simulink model "reactorBlock_Simulink_Simscape_Full_Controller"  (R2023a)
settings: Solver=ode15s  StartTime=0.0  StopTime=300  FixedStep=0.1  RelTol=1e-3
libraries: nesl_utility x30, fl_lib x28, slpidlib x4, simulink x4, RankineCycle_lib x3
(part 2 of 2)

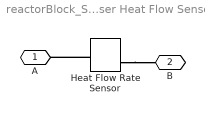
== system reactorBlock_Simulink_Simscape_Full_Controller/Condenser Heat Flow Sensor ==
  Heat Flow Rate Sensor : fl_lib/Thermal/Thermal Sensors/Heat Flow Rate Sensor
  A : PMIOPort  Side=Left
  B : PMIOPort  Port=2  Side=Right
  connections:
  Heat Flow Rate Sensor/RConn2 -- B/RConn1
  Heat Flow Rate Sensor/LConn1 -- A/RConn1
